simulink model "plantMRUE5"  (R2023b)
settings: Solver=VariableStepAuto  StartTime=0.0  StopTime=7  RelTol=1e-3
model workspace (MATLAB code in the model file):
  | %% True Parameters
  | % Masses
  | mw=0.1;
  | mb=1;
  | M=1.2;
  | 
  | % Distances
  | rho=0.07;
  | l=0.02;
  | d=0.015; % distance A-C
  | 
  | % Electriques
  | L=1e-3;
  | R=1e-1;
  | % r;
  | 
  | % Couples
  | k=1e-2;
  | % alpha=34.6;
  | % beta=2.06e5;
  | 
  | % Moments inertie
  | Iwy=2.45e-4;
  | Ipsi=1.53e-2;
  | 
  | % Utilitaire
  | beta = (M + 2*Iwy/rho^2);
  | gamma = Ipsi + mb*d^2;
  | 
  | %% Nominal Equilibrium Trajectory: Horizontal MRU
  | 
  | % We command speed
  | uref = 1; %m/s
  | psiref = 0;
  | 
  | Usbar = min([2*k/rho*uref; 12]); % should not be >12V
  | 
  | Urbar = Usbar/2; %right
  | Ulbar = Usbar/2;
  | 
  | %% Slow State
  | pbar = 0; % is not in state function, any value fits
  | % normally, should equals ubar*t.
  | ubar = uref;
  | psibar = psiref;
  | vbar = 0;
  | xbar = pbar;
  | ybar = 0;
  | 
  | % IMPORTANT: following only true at t=0s.
  | slowstatebar = [pbar; ubar; psibar; vbar; xbar; ybar];
  | 
  | 
  | %% Fast State
  | irbar = 0;
  | ilbar = 0;
  | 
  | faststatebar = [irbar; ilbar];
settings Model: Creator=Jules  LastModifiedBy=Jules

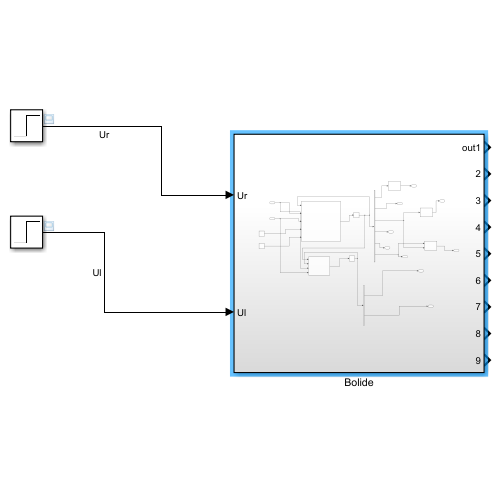
[thumbnail: Simulink's stored preview of the top-level diagram]
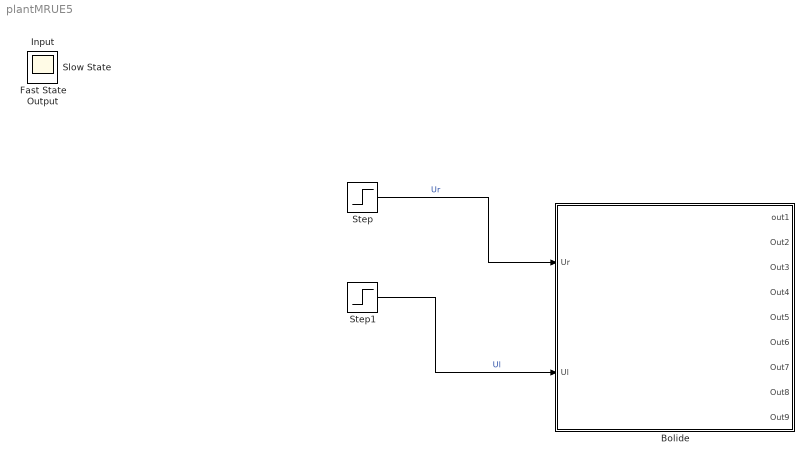
== system plantMRUE5 ==
  Bolide : Subsystem
  Step : Step  Time=5  Before=Urbar  After=Urbar  SampleTime=0
  Step1 : Step  Time=2  Before=Ulbar  After=Ulbar  SampleTime=0
  Fast State : Scope
  Input : Scope
  Output : Scope
  Slow State : Scope
  wires:
  Step/1 -> Bolide/1(Ur)  "Ur"
  Step1/1 -> Bolide/2(Ul)  "Ul"

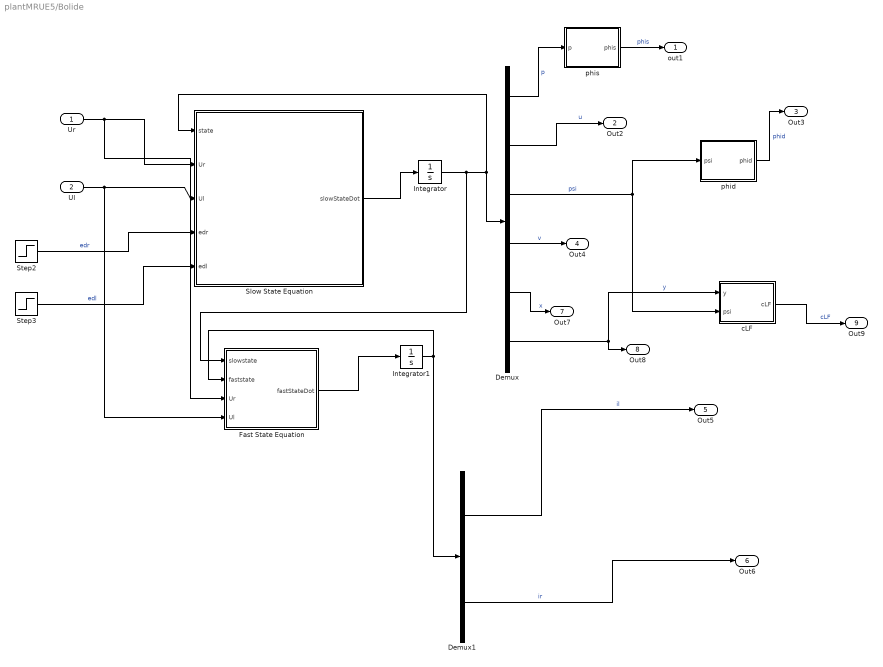
== system plantMRUE5/Bolide ==
  Ur : Inport
  Ul : Inport  Port=2
  Demux : Demux  Outputs=6
  Demux1 : Demux  Outputs=2
  Fast State Equation : MATLAB Function  TreatAsAtomicUnit=on
  Integrator : Integrator  InitialCondition=slowstatebar
  Integrator1 : Integrator  InitialCondition=faststatebar
  Slow State Equation : MATLAB Function  TreatAsAtomicUnit=on
  Step2 : Step  After=0  SampleTime=0
  Step3 : Step  After=0  SampleTime=0
  cLF : MATLAB Function  TreatAsAtomicUnit=on
  phid : MATLAB Function  TreatAsAtomicUnit=on
  phis : MATLAB Function  TreatAsAtomicUnit=on
  out1 : Outport
  Out2 : Outport  Port=2
  Out3 : Outport  Port=3
  Out4 : Outport  Port=4
  Out5 : Outport  Port=5
  Out6 : Outport  Port=6
  Out7 : Outport  Port=7
  Out8 : Outport  Port=8
  Out9 : Outport  Port=9
  wires:
  Step3/1 -> Slow State Equation/5(edl)  "edl"
  Slow State Equation/1(slowStateDot) -> Integrator/1
  Integrator/1 -> Fast State Equation/1(slowstate), Slow State Equation/1(state), Demux/1
  Step2/1 -> Slow State Equation/4(edr)  "edr"
  Ul/1 -> Fast State Equation/4(Ul), Slow State Equation/3(Ul)
  Ur/1 -> Fast State Equation/3(Ur), Slow State Equation/2(Ur)
  Demux/1 -> phis/1(p)  "p"
  Demux/6 -> Out8/1, cLF/1(y)  "y"
  Demux/5 -> Out7/1  "x"
  Demux/2 -> Out2/1  "u"
  Demux1/2 -> Out6/1  "ir"
  Demux/4 -> Out4/1  "v"
  Demux1/1 -> Out5/1  "il"
  phis/1(phis) -> out1/1  "phis"
  Demux/3 -> phid/1(psi), cLF/2(psi)  "psi"
  phid/1(phid) -> Out3/1  "phid"
  cLF/1(cLF) -> Out9/1  "cLF"
  Fast State Equation/1(fastStateDot) -> Integrator1/1
  Integrator1/1 -> Fast State Equation/2(faststate), Demux1/1

== matlab function plantMRUE5/Bolide/cLF ==
  data: y input; cLF output; psi input; psibar parameter; ybar parameter
function cLF = fcn(y, psi, psibar, ybar)

cLF = y/cos(psi - psibar);

== matlab function plantMRUE5/Bolide/Slow State Equation ==
  data: state input; slowStateDot output; Ur input; Ul input; edr input; edl input; M parameter; rho parameter; l parameter; Iwy parameter; Ipsi parameter; d parameter; L parameter; R parameter; k parameter; mb parameter; beta parameter; gamma parameter
function slowStateDot = fcn(state,Ur, Ul, edr, edl, M, rho, l, Iwy, Ipsi, d, L, R, k, mb, beta, gamma)
% ed est l'entrée de perturbation, != d (distance AC)
% Model parameters M,Ipsi,d,L,R,k defined in "Model Explorer/Matlab Code"

%% Système Lent
p = state(1); % intégrale temporelle de u, distance parcourue
u = state(2);
psi = state(3);
v = state(4); % psidot
x = state(5); % ordonnée point A
y = state(6); % abscisse point A

Us = Ur + Ul + edr + edl;
Ud = Ur - Ul + edr - edl;

pdot = u;
udot = k/rho/beta/R*Us - 2*k^2/beta/rho^2/R*u - mb*d/beta*v^2;
psidot = v;
vdot = l*k/2/gamma/R/rho*Ud - k^2*l^2/2/gamma/rho^2/R*v + mb*d/gamma*u*v;
xdot = cos(psi)*u;
ydot = sin(psi)*u;

slowStateDot = [pdot; udot; psidot; vdot; xdot; ydot];

== matlab function plantMRUE5/Bolide/phid ==
  data: psi input; phid output; rho parameter; l parameter
function phid = fcn(psi, rho, l)

phid = l/rho*psi;

== matlab function plantMRUE5/Bolide/phis ==
  data: rho parameter; p input; phis output
function phis = fcn(rho,p)

phis = 2/rho*p;

== matlab function plantMRUE5/Bolide/Fast State Equation ==
  data: slowstate input; faststate input; Ur input; Ul input; R parameter; fastStateDot output; L parameter; k parameter; rho parameter; l parameter
function fastStateDot = fcn(slowstate,faststate,Ur,Ul,R,L,k,rho, l)
%% Système Rapide

u = slowstate(2);
v = slowstate(4);
ir = faststate(1); % Intensité à gauche
il = faststate(2);

is = ir + il; % Somme
id = ir - il; % Diff
Us = Ur + Ul;
Ud = Ur - Ul;

isdot = 1/L*(Us - R*is - 2*k/rho*u);
iddot = 1/L*(Ud - R*id - k*l/rho*v);

irdot = 0.5*(isdot + iddot); % droite
ildot = 0.5*(isdot - iddot);

fastStateDot=[irdot; ildot];
